simulink model "magnent"  (R2017a)
settings: Solver=FixedStepAuto  StartTime=0.0  StopTime=10.0  FixedStep=0.001  RelTol=1e-3
settings Model: Creator=Administrator  LastModifiedBy=Administrator

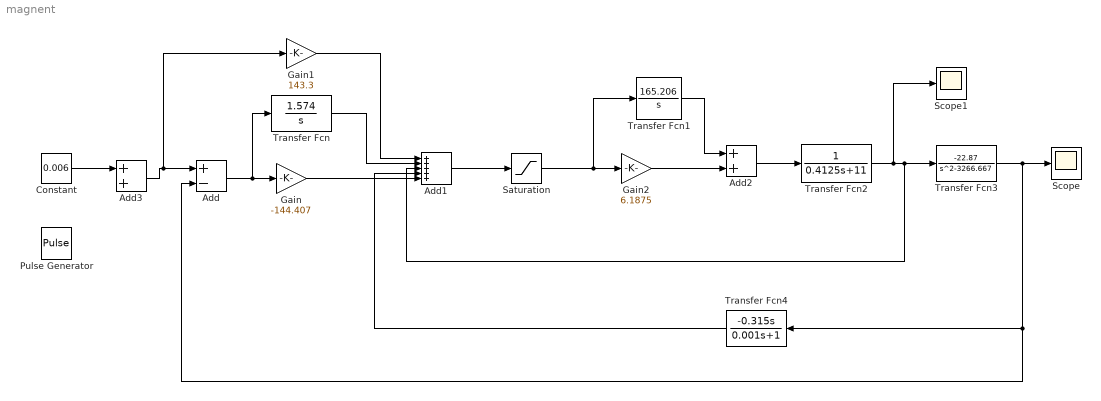
== system magnent ==
  Add : Sum  Inputs=+-
  Add1 : Sum  Inputs=+++++
  Add2 : Sum
  Add3 : Sum
  Constant : Constant  Value=0.006
  Gain : Gain  Gain=-144.407
  Gain1 : Gain  Gain=143.3
  Gain2 : Gain  Gain=6.1875
  Pulse Generator : DiscretePulseGenerator  PulseType=Time based  Amplitude=0.001  Period=10  PulseWidth=5
  Saturation : Saturate  UpperLimit=3  LowerLimit=-3
  Scope : Scope
  Scope1 : Scope
  Transfer Fcn : TransferFcn  Numerator=[1.574]  Denominator=[1 0]
  Transfer Fcn1 : TransferFcn  Numerator=[165.206]  Denominator=[1 0]
  Transfer Fcn2 : TransferFcn  Denominator=[0.4125 11]
  Transfer Fcn3 : TransferFcn  Numerator=[-22.87]  Denominator=[1 0 -3266.667]
  Transfer Fcn4 : TransferFcn  Numerator=[-0.315 0]  Denominator=[0.001 1]
  wires:
  Add/1 -> Transfer Fcn/1, Gain/1
  Gain/1 -> Add1/3
  Transfer Fcn/1 -> Add1/2
  Gain1/1 -> Add1/1
  Gain2/1 -> Add2/2
  Transfer Fcn1/1 -> Add2/1
  Add2/1 -> Transfer Fcn2/1
  Transfer Fcn3/1 -> Transfer Fcn4/1, Add/2, Scope/1
  Transfer Fcn4/1 -> Add1/4
  Transfer Fcn2/1 -> Scope1/1, Add1/5, Transfer Fcn3/1
  Constant/1 -> Add3/1
  Add3/1 -> Gain1/1, Add/1
  Add1/1 -> Saturation/1
  Saturation/1 -> Transfer Fcn1/1, Gain2/1
